simulink model "IoTSimulationFinal"  (R2021a)
settings: Solver=VariableStepAuto  StartTime=0.0  StopTime=100.0  RelTol=1e-3
libraries: simulink x4, spsSawtoothGeneratorLib x2, spsStairGeneratorLib x1
settings Model: Creator=user  LastModifiedBy=user

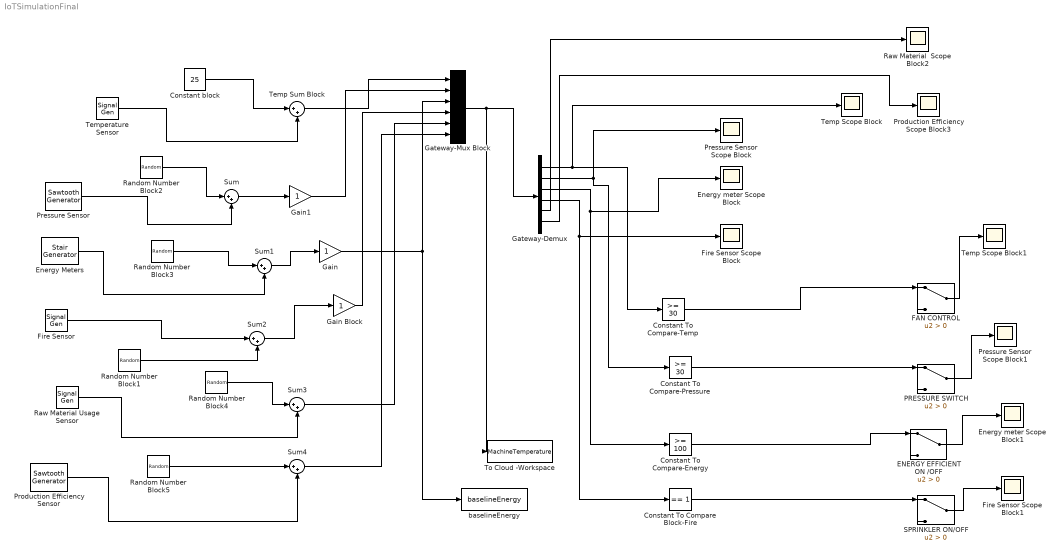
== system IoTSimulationFinal ==
  Constant To Compare Block-Fire : simulink/Logic and Bit Operations/Compare To Constant  relop===  const=1  OutDataTypeStr=boolean
  Constant To Compare-Energy : simulink/Logic and Bit Operations/Compare To Constant  relop=>=  const=100  OutDataTypeStr=boolean
  Constant To Compare-Pressure : simulink/Logic and Bit Operations/Compare To Constant  relop=>=  const=30  OutDataTypeStr=boolean
  Constant To Compare-Temp : simulink/Logic and Bit Operations/Compare To Constant  relop=>=  const=30  OutDataTypeStr=boolean
  Constant block : Constant  Value=25
  ENERGY EFFICIENT ON /OFF : Switch  Criteria=u2 > Threshold
  Energy Meters : spsStairGeneratorLib/Stair Generator  t=[0, 1, 3, 3.5]  e=[1, -1, 2.5, 0]  Ts=0
  Energy meter Scope Block : Scope
  Energy meter Scope Block1 : Scope
  FAN CONTROL : Switch  Criteria=u2 > Threshold
  Fire Sensor : SignalGenerator  WaveForm=square  Units=rad/sec
  Fire Sensor Scope Block : Scope
  Fire Sensor Scope Block1 : Scope
  Gain : Gain
  Gain Block : Gain
  Gain1 : Gain
  Gateway-Demux : Demux  Outputs=6
  Gateway-Mux Block : Mux  Inputs=6
  PRESSURE SWITCH : Switch  Criteria=u2 > Threshold
  Pressure Sensor : spsSawtoothGeneratorLib/Sawtooth Generator  Freq=1e3  Phase=180  Ts=0
  Pressure Sensor Scope Block : Scope
  Pressure Sensor Scope Block1 : Scope
  Production Efficiency Scope Block3 : Scope
  Production Efficiency Sensor : spsSawtoothGeneratorLib/Sawtooth Generator  Freq=1e3  Phase=180  Ts=0
  Random Number Block1 : RandomNumber  Variance=0.1  SampleTime=0.1
  Random Number Block{2..5} (4 alike) : RandomNumber  SampleTime=0.1
  Raw Material  Scope Block2 : Scope
  Raw Material Usage Sensor : SignalGenerator  Amplitude=10  Units=rad/sec
  SPRINKLER ON/OFF : Switch  Criteria=u2 > Threshold
  Sum{,1..4} (5 alike) : Sum  Inputs=|++
  Temp Scope Block : Scope
  Temp Scope Block1 : Scope
  Temp Sum Block : Sum  Inputs=|++
  Temperature Sensor : SignalGenerator  Amplitude=10  Units=rad/sec
  To Cloud -Workspace : ToWorkspace  VariableName=MachineTemperature  SaveFormat=Structure With Time  SampleTime=-1
  baselineEnergy : ToWorkspace  VariableName=baselineEnergy  SaveFormat=Structure With Time  SampleTime=-1
  wires:
  Temperature Sensor/1 -> Temp Sum Block/2
  Temp Sum Block/1 -> Gateway-Mux Block/1
  Pressure Sensor/1 -> Sum/2
  Sum/1 -> Gain1/1
  Random Number Block1/1 -> Sum2/2
  Fire Sensor/1 -> Sum2/1
  Sum2/1 -> Gain Block/1
  Random Number Block2/1 -> Sum/1
  Energy Meters/1 -> Sum1/2
  Sum1/1 -> Gain/1
  Random Number Block3/1 -> Sum1/1
  Gain1/1 -> Gateway-Mux Block/2
  Gain/1 -> baselineEnergy/1, Gateway-Mux Block/3
  Gain Block/1 -> Gateway-Mux Block/4
  Constant block/1 -> Temp Sum Block/1
  Gateway-Mux Block/1 -> Gateway-Demux/1, To Cloud -Workspace/1
  Constant To Compare Block-Fire/1 -> SPRINKLER ON/OFF/1
  Constant To Compare-Temp/1 -> FAN CONTROL/1
  Constant To Compare-Energy/1 -> ENERGY EFFICIENT ON /OFF/1
  Constant To Compare-Pressure/1 -> PRESSURE SWITCH/1
  Gateway-Demux/1 -> Temp Scope Block/1, Constant To Compare-Temp/1
  Gateway-Demux/4 -> Constant To Compare Block-Fire/1, Fire Sensor Scope Block/1
  Gateway-Demux/2 -> Constant To Compare-Pressure/1, Pressure Sensor Scope Block/1
  Gateway-Demux/3 -> Constant To Compare-Energy/1, Energy meter Scope Block/1
  FAN CONTROL/1 -> Temp Scope Block1/1
  PRESSURE SWITCH/1 -> Pressure Sensor Scope Block1/1
  ENERGY EFFICIENT ON /OFF/1 -> Energy meter Scope Block1/1
  SPRINKLER ON/OFF/1 -> Fire Sensor Scope Block1/1
  Random Number Block4/1 -> Sum3/1
  Random Number Block5/1 -> Sum4/1
  Production Efficiency Sensor/1 -> Sum4/2
  Raw Material Usage Sensor/1 -> Sum3/2
  Sum3/1 -> Gateway-Mux Block/5
  Sum4/1 -> Gateway-Mux Block/6
  Gateway-Demux/5 -> Raw Material  Scope Block2/1
  Gateway-Demux/6 -> Production Efficiency Scope Block3/1
